simulink model "paper_two_inertia_system"  (R2022b)
settings: Solver=VariableStepAuto  StartTime=0.0  StopTime=1000  RelTol=1e-14
settings Model: Creator=saayu  LastModifiedBy=saayu

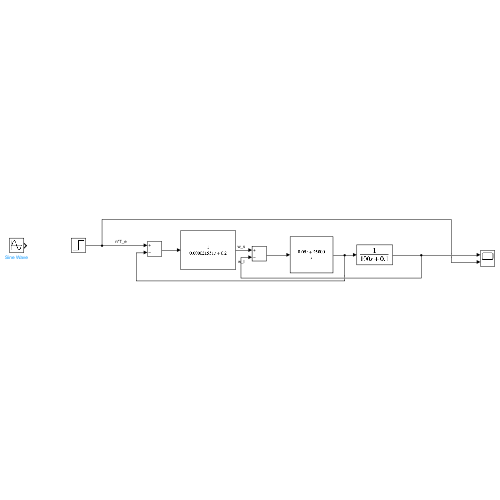
[thumbnail: Simulink's stored preview of the top-level diagram]
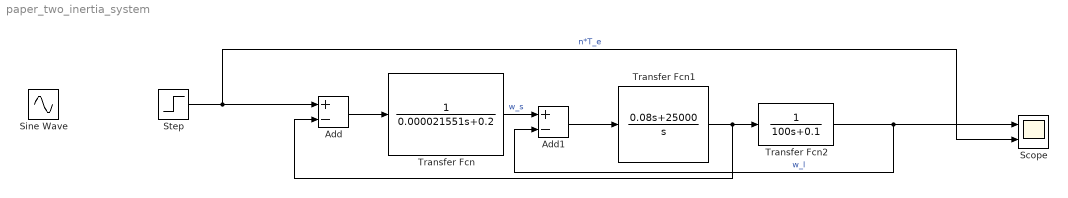
== system paper_two_inertia_system ==
  Add : Sum  Inputs=+-
  Add1 : Sum  Inputs=+-
  Scope : Scope  NumInputPorts=2
  Sine Wave : Sin  Amplitude=1000  Frequency=0.1  SampleTime=0
  Step : Step  Time=20  After=100  SampleTime=0
  Transfer Fcn : TransferFcn  Denominator=[0.000021551 0.2]
  Transfer Fcn1 : TransferFcn  Numerator=[0.08 25000]  Denominator=[1 0]
  Transfer Fcn2 : TransferFcn  Denominator=[100 0.1]
  wires:
  Transfer Fcn2/1 -> Add1/2, Scope/1  "w_l"
  Transfer Fcn1/1 -> Add/2, Transfer Fcn2/1
  Step/1 -> Scope/2, Add/1  "n*T_e"
  Add/1 -> Transfer Fcn/1
  Transfer Fcn/1 -> Add1/1  "w_s"
  Add1/1 -> Transfer Fcn1/1
